simulink model "IP02_FreqTest"  (R2024b)
settings: Solver=ode45  StartTime=0.0  StopTime=120  MaxStep=1e-3  RelTol=1e-4  AbsTol=1e-6
settings Model: Creator=Karim Negm  LastModifiedBy=Karim Negm

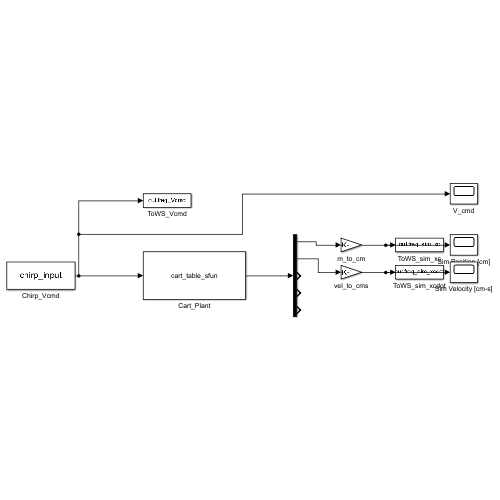
[thumbnail: Simulink's stored preview of the top-level diagram]
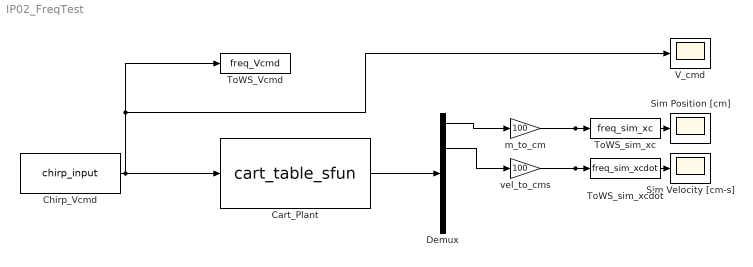
== system IP02_FreqTest ==
  Cart_Plant : M-S-Function  FunctionName=cart_table_sfun
  Chirp_Vcmd : FromWorkspace  VariableName=chirp_input
  Demux : Demux  Outputs=5
  Sim Position [cm] : Scope
  Sim Velocity [cm-s] : Scope
  ToWS_Vcmd : ToWorkspace  VariableName=freq_Vcmd  SaveFormat=Timeseries  SampleTime=-1
  ToWS_sim_xc : ToWorkspace  VariableName=freq_sim_xc  SaveFormat=Timeseries  SampleTime=-1
  ToWS_sim_xcdot : ToWorkspace  VariableName=freq_sim_xcdot  SaveFormat=Timeseries  SampleTime=-1
  V_cmd : Scope
  m_to_cm : Gain  Gain=100
  vel_to_cms : Gain  Gain=100
  wires:
  Chirp_Vcmd/1 -> V_cmd/1, ToWS_Vcmd/1, Cart_Plant/1
  Cart_Plant/1 -> Demux/1
  Demux/1 -> m_to_cm/1
  Demux/2 -> vel_to_cms/1
  m_to_cm/1 -> Sim Position [cm]/1, ToWS_sim_xc/1
  vel_to_cms/1 -> Sim Velocity [cm-s]/1, ToWS_sim_xcdot/1
